simulink model "slrt_induction_2level_inverter"  (R2022b)
settings: Solver=FixedStepAuto  StartTime=0.0  StopTime=0.25  RelTol=1e-3  EnableMultiTasking=on
PreLoadFcn:
  | Ts = 1e-4;
  | Tcpu = 50e-6; %Controller sample time
  | 
  | % PMSM parameters
  | PM = 0.03; % Permanent magnet flux linkage
  | Ld = 2e-4;  % d-axis inductance
  | Lq = 2e-4;  % q-axis inductance
  | L0 = 2e-4;  % 0-axis inductance
  | Rs = 0.013; % Stator resistance
  | N = 6; % Number of pole pairs
  | J = 0.2; % Moment of inertia
  | 
  | % encoder parameters
  | numSlits = 2000; % number of slits
  | pulseSigOffset = 0; % index pulse signal offset
  | shaftInitPos = 0; % motor shaft initial position
  | 
  | % DAC parameters
  | gain = 0.1;
  | bias = 0;
  | 
  | % circuit parameters
  | Vdc = 48;
  | 
  | % real-time parameters
  | ts_FPGA_clk = 5e-9;
  | ts_FPGA_mdl = 1e-6;
  | 
  | % Real-time processor or embedded controller
  | RTorTTL = 1; % 1: Real-time processor,    0: embedded controller
  | 
  | % sample times
  | f_base = 200e6;
  | PWM_frequency = 20e3;
  | ts_FPGA_clk = 1/f_base;
  | ts_FPGA_mdl =1e-6;
undefined symbols (not defined in the file or in its folder): DiscIntNeverNeededParam
libraries: simulink x7, hdlsllib x3, slrtencoderlib x2, slrtresolverlib x2, mcbhdlplantlib x1, slrthdlutillib x1, slrt2levelinverterlib x1
(part 2 of 2)

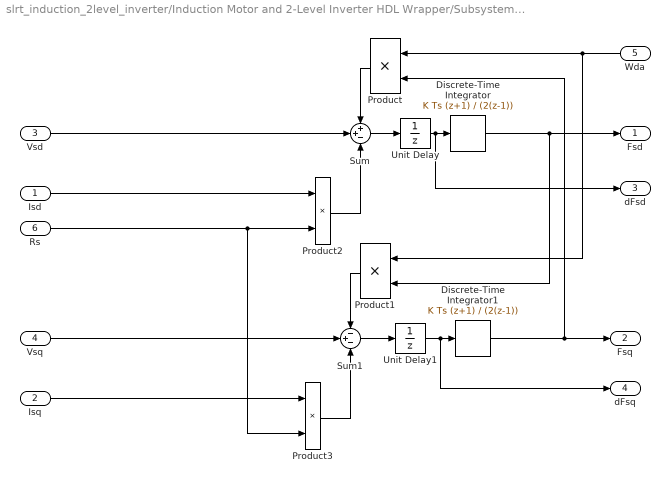
== system slrt_induction_2level_inverter/Induction Motor and 2-Level Inverter HDL Wrapper/Subsystem/Induction Motor HDL/IM HDL/IM Electromagnetic Discrete/IM Equivalent Circuit/Stator Flux ==
  Isd : Inport
  Isq : Inport  Port=2
  Vsd : Inport  Port=3
  Vsq : Inport  Port=4
  Wda : Inport  Port=5
  Rs : Inport  Port=6
  Discrete-Time Integrator : DiscreteIntegrator  IntegratorMethod=Integration: Trapezoidal  SampleTime=Ts  RndMeth=Simplest  ICPrevOutput=DiscIntNeverNeededParam  ICPrevScaledInput=DiscIntNeverNeededParam
  Discrete-Time Integrator1 : DiscreteIntegrator  IntegratorMethod=Integration: Trapezoidal  SampleTime=Ts  RndMeth=Simplest  ICPrevOutput=DiscIntNeverNeededParam  ICPrevScaledInput=DiscIntNeverNeededParam
  Product : Product  InputSameDT=on  RndMeth=Simplest  SaturateOnIntegerOverflow=on  OutDataTypeStr=Inherit: Same as first input
  Product1 : Product  InputSameDT=on  RndMeth=Simplest  SaturateOnIntegerOverflow=on  OutDataTypeStr=Inherit: Same as first input
  Product2 : Product  RndMeth=Simplest  OutDataTypeStr=Inherit: Same as first input
  Product3 : Product  RndMeth=Simplest  OutDataTypeStr=Inherit: Same as first input
  Sum : Sum  Inputs=++-  InputSameDT=on  SaturateOnIntegerOverflow=on  OutDataTypeStr=Inherit: Same as first input
  Sum1 : Sum  Inputs=-+-  InputSameDT=on  RndMeth=Simplest  SaturateOnIntegerOverflow=on  OutDataTypeStr=Inherit: Same as first input
  Unit Delay : UnitDelay  SampleTime=-1  HasFrameUpgradeWarning=on
  Unit Delay1 : UnitDelay  SampleTime=-1  HasFrameUpgradeWarning=on
  Fsd : Outport  VectorParamsAs1DForOutWhenUnconnected=off
  Fsq : Outport  Port=2  VectorParamsAs1DForOutWhenUnconnected=off
  dFsd : Outport  Port=3  VectorParamsAs1DForOutWhenUnconnected=off
  dFsq : Outport  Port=4  VectorParamsAs1DForOutWhenUnconnected=off
  wires:
  Discrete-Time Integrator/1 -> Fsd/1, Product1/2
  Discrete-Time Integrator1/1 -> Fsq/1, Product/2
  Unit Delay1/1 -> Discrete-Time Integrator1/1, dFsq/1
  Unit Delay/1 -> Discrete-Time Integrator/1, dFsd/1
  Rs/1 -> Product2/2, Product3/2
  Product3/1 -> Sum1/3
  Isq/1 -> Product3/1
  Vsq/1 -> Sum1/2
  Product1/1 -> Sum1/1
  Sum1/1 -> Unit Delay1/1
  Product2/1 -> Sum/3
  Isd/1 -> Product2/1
  Vsd/1 -> Sum/2
  Wda/1 -> Product/1, Product1/1
  Product/1 -> Sum/1
  Sum/1 -> Unit Delay/1
